simulink library "ground_storage_U_tube"  (Simulink 8.2)
settings: Solver=ode45  StartTime=0.0  StopTime=10.0  RelTol=1e-3
libraries: carnot x3
settings Model: Creator=lena.frank  LastModifiedBy=ralf.dott

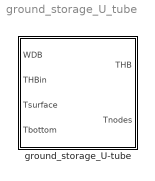
== system ground_storage_U_tube ==
  ground_storage_U-tube : Subsystem  InitFcn=disp('ATTENTION: MODEL ground_storage_U-tube IS NOT VALIDATED !')  mask(borehole ground storage){ds=1, hs=1, dh=0.05, hh=1, ground=clay (humid), borehole=clay (humid), dp=0.02, kp=0.001, t0=10, rn=6, zn=6, mpts=3}
      mask prompts: ds "diameter of storage region [m]"; hs "depth of storage region [m]"; dh "diameter of borehole [m]"; hh "depth of borehole [m]"; borehole "borehole filling"; dp "diameter of pipe [m]"; kp "roughness of pipe [m]"; t0 "initial temperature [degree centigrade]"; rn "number of radial nodes"; zn "number of axial nodes"; mpts "number of measurement points"
      mask help:
      | Model for the calculation of an U-tube ground storage.
      | Look under mask to change the surface model.
      |
      | ATTENTION: MODEL IS NOT VALIDATED !
      mask init:
      | ds = max(ds, 0.001);
      | hs = max(hs, 0.001);
      | dh = max(dh, 0.001);
      | hh = min(hs, max(hh, 0.001));
      | cond=[0.7 1.88 1.45 2.9 0.58];
      | le = cond(ground);
      | cap = [1382400 1798200 2410560 2864160 1798200];
      | ce = cap(ground);
      | lh = cond(borehole);
      | ch = cap(borehole);
      mask Help: web(fullfile(path_carnot('help'),'ground_storage_U_tube.html'),'-helpbrowser')
      mask TypeOptions ground: sand (dry) | sand (saturated with water) | clay (humid) | clay (saturated with water)
      mask TypeOptions borehole: sand (dry) | sand (saturated with water) | clay (humid) | clay (saturated with water) | bentonit (83% water)
      mask Display: plot(0,10,100,90,[70,30],[80,80],[35,35,43,43,47,52,57,57,66,66,60,60,54,46,40,40,35],[84,87,87,20,13,13,21,87,87,84,84,20,10,10,20,84,84])

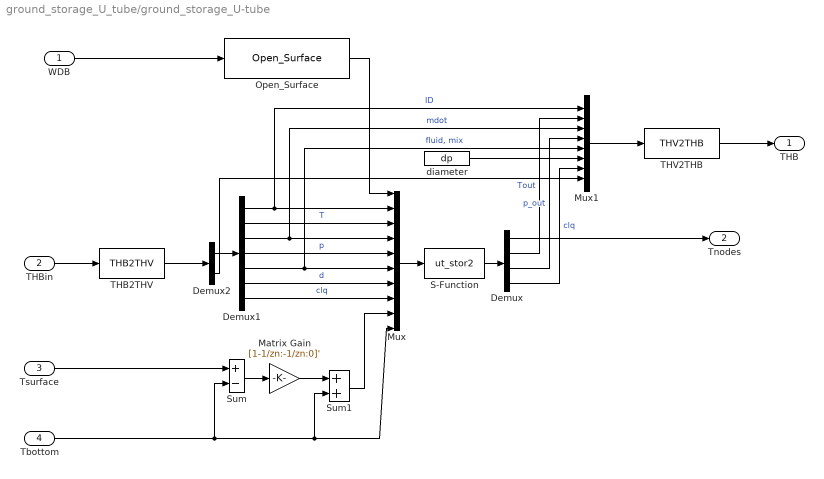
== system ground_storage_U_tube/ground_storage_U-tube ==
  WDB : Inport
  THBin : Inport  Port=2
  Tsurface : Inport  Port=3
  Tbottom : Inport  Port=4
  Demux : Demux  Outputs=[3*mpts 1 1 3]
  Demux1 : Demux  Outputs=[1 1 1 1 2 1 3]
  Demux2 : Demux  Outputs=[10 10]
  Matrix Gain : Gain  Gain=[1-1/zn:-1/zn:0]'  SaturateOnIntegerOverflow=on  OutDataTypeStr=Inherit: Same as input  ParamDataTypeStr=Inherit: Same as input
  Mux : Mux  Inputs=10
  Mux1 : Mux  Inputs=8
  Open_Surface : carnot/Storage/Thermal/surface_models/Open_Surface  albedo=0.6
  S-Function : S-Function  FunctionName=ut_stor2  Parameters=ds, hs, ce, le, dp, dh, hh, ch, lh, kp, t0, rn, zn, mpts  EnableBusSupport=off
  Sum : Sum  Inputs=+-  SaturateOnIntegerOverflow=on  InputSameDT=on  OutDataTypeStr=Inherit: Same as first input
  Sum1 : Sum  SaturateOnIntegerOverflow=on  InputSameDT=on  OutDataTypeStr=Inherit: Same as first input
  THB2THV : carnot/Toolbox/THB2THV
  THV2THB : carnot/Toolbox/THV2THB
  diameter : Constant  Value=dp
  THB : Outport
  Tnodes : Outport  Port=2
  wires:
  THV2THB/1 -> THB/1
  THB2THV/1 -> Demux2/1
  Tbottom/1 -> Sum1/2, Mux/10, Sum/2
  Matrix Gain/1 -> Sum1/1
  Sum/1 -> Matrix Gain/1
  Tsurface/1 -> Sum/1
  Demux1/5 -> Mux1/5, Mux/6  "fluid, mix"
  Demux1/3 -> Mux1/3, Mux/4  "mdot"
  Demux1/6 -> Mux/7  "d"
  Demux1/4 -> Mux/5  "p"
  Demux1/2 -> Mux/3  "T"
  Mux/1 -> S-Function/1
  Demux1/1 -> Mux1/1, Mux/2  "ID"
  Open_Surface/1 -> Mux/1
  Demux2/1 -> Demux1/1
  THBin/1 -> THB2THV/1
  Demux2/2 -> Mux1/8
  diameter/1 -> Mux1/6
  WDB/1 -> Open_Surface/1
  S-Function/1 -> Demux/1
  Demux/3 -> Mux1/4  "p_out"
  Demux/2 -> Mux1/2  "Tout"
  Sum1/1 -> Mux/9
  Demux1/7 -> Mux/8  "clq"
  Demux/4 -> Mux1/7  "clq"
  Demux/1 -> Tnodes/1
  Mux1/1 -> THV2THB/1
